simulink model "mm_simplerobot"  (R2025b)
settings: Solver=ode3  StartTime=0.0  StopTime=inf  FixedStep=0.01  RelTol=1e-3
libraries: mmuct_lib x2
settings Model: Creator=nicolls  LastModifiedBy=nicolls
settings OptimizationCC: BlockReduction=off

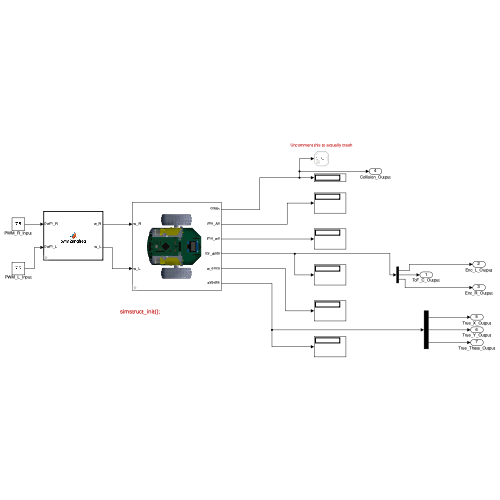
[thumbnail: Simulink's stored preview of the top-level diagram]
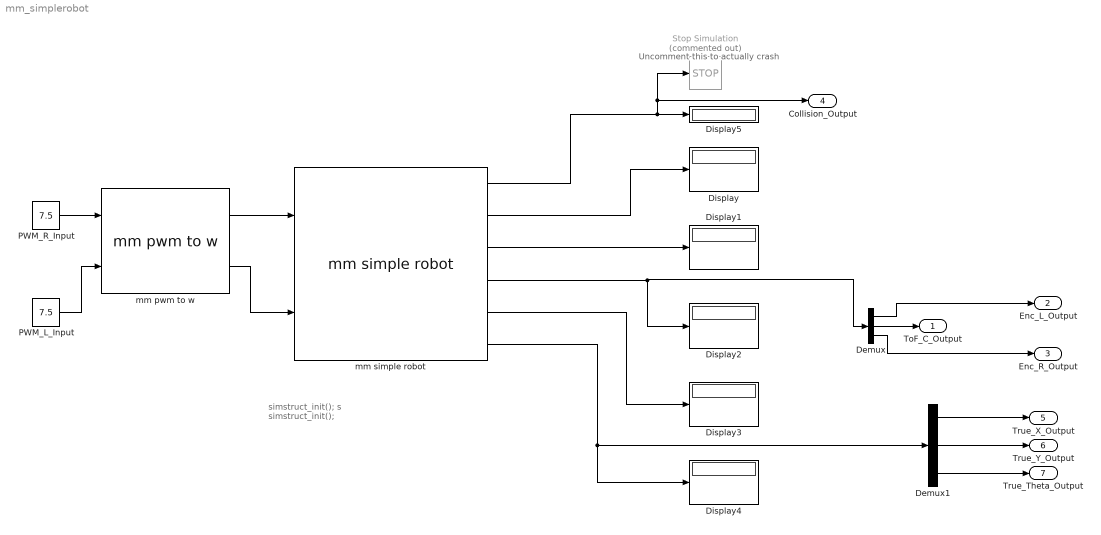
== system mm_simplerobot ==
  note: Uncomment this to actually crash
  note: simstruct_init();
      | s
      | simstruct_init();
  Demux : Demux  Outputs=3
  Demux1 : Demux  Outputs=3
  Display{,1..5} (6 alike) : Display
  PWM_L_Input : Constant  Value=7.5
  PWM_R_Input : Constant  Value=7.5
  Stop Simulation : Stop  Commented=on
  mm pwm to w : mmuct_lib/mm pwm to w  deadb=0  maxw=2*pi  motd=0
  mm simple robot : mmuct_lib/mm simple robot  simstruct=simstruct  x0=0.1  y0=0.1  theta0=0
  ToF_C_Output : Outport
  Enc_L_Output : Outport  Port=2
  Enc_R_Output : Outport  Port=3
  Collision_Output : Outport  Port=4
  True_X_Output : Outport  Port=5
  True_Y_Output : Outport  Port=6
  True_Theta_Output : Outport  Port=7
  wires:
  mm simple robot/1 -> Stop Simulation/1, Collision_Output/1, Display5/1
  mm simple robot/2 -> Display/1
  mm simple robot/3 -> Display1/1
  mm simple robot/4 -> Display2/1, Demux/1
  PWM_R_Input/1 -> mm pwm to w/1
  PWM_L_Input/1 -> mm pwm to w/2
  Demux/2 -> ToF_C_Output/1
  Demux/1 -> Enc_L_Output/1
  Demux/3 -> Enc_R_Output/1
  mm pwm to w/1 -> mm simple robot/1
  mm pwm to w/2 -> mm simple robot/2
  mm simple robot/5 -> Display3/1
  mm simple robot/6 -> Demux1/1, Display4/1
  Demux1/1 -> True_X_Output/1
  Demux1/2 -> True_Y_Output/1
  Demux1/3 -> True_Theta_Output/1
